simulink model "RLC_devresi"  (Simulink 10.1)
settings: Solver=VariableStepAuto  StartTime=0.0  StopTime=stopTime  RelTol=1e-3
values from neighbouring files (symbols this model uses):
  C = 0.01    [init_RLC_devresi.m]
  L = 1    [init_RLC_devresi.m]
  R = 0    [init_RLC_devresi.m]
  Vcc = 5    [RC_dogal_cevap.m]    (also in RC_zorlanmis_cevap.m; RL_dogal_cevap.m; RL_zorlanmis_cevap.m; init_RLC_devresi.m)
settings Model: Creator=TULPAR  LastModifiedBy=TULPAR
settings DataIOCC: SaveFormat=Dataset  ReturnWorkspaceOutputs=on
settings OptimizationCC: LifeSpan=auto
settings DebuggingCC: UnderspecifiedInitializationDetection=Simplified  MergeDetectMultiDrivingBlocksExec=error  SFUnexpectedBacktrackingDiag=error  SFNoUnconditionalDefaultTransitionDiag=error  SFExecutionAtInitializationDiag=warning  ArithmeticOperatorsInVariantConditions=error
settings HardwareCC: ProdBitPerPointer=64  ProdBitPerSizeT=64  ProdBitPerPtrDiffT=64  ProdLargestAtomicFloat=Float  ProdIntDivRoundTo=Zero  ProdEndianess=LittleEndian  ProdWordSize=64  ProdHWDeviceType=Intel->x86-64 (Windows64)
settings ModelReferenceCC: PropagateSignalLabelsOutOfModel=on
settings SFSimCC: SimUseLocalCustomCode=on  CustomCodeUndefinedFunction=FilterOut
settings RTWCC: RTWUseLocalCustomCode=on
settings CodeAppCC: StateflowObjectComments=off
settings GRTTargetCC: TargetLangStandard=C99 (ISO)  CombineOutputUpdateFcns=on  GRTInterface=off
settings ConfigComp: CovMetricSettings=dwe  CovHtmlReporting=off  CovSaveCumulativeToWorkspaceVar=off  CovSaveSingleToWorkspaceVar=off  CovExternalEMLEnable=on

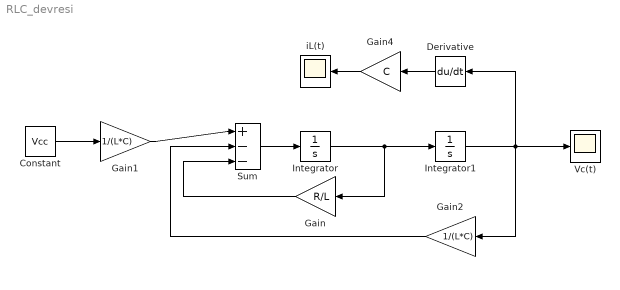
== system RLC_devresi ==
  Constant : Constant  Value=Vcc
  Derivative : Derivative
  Gain : Gain  Gain=R/L
  Gain1 : Gain  Gain=1/(L*C)
  Gain2 : Gain  Gain=1/(L*C)
  Gain4 : Gain  Gain=C
  Integrator : Integrator
  Integrator1 : Integrator
  Sum : Sum  Inputs=|+--
  Vc(t) : Scope
  iL(t) : Scope
  wires:
  Integrator/1 -> Integrator1/1, Gain/1
  Constant/1 -> Gain1/1
  Gain1/1 -> Sum/1
  Gain2/1 -> Sum/2
  Gain/1 -> Sum/3
  Sum/1 -> Integrator/1
  Integrator1/1 -> Vc(t)/1, Derivative/1, Gain2/1
  Derivative/1 -> Gain4/1
  Gain4/1 -> iL(t)/1
